simulink model "R2RSystemModel"  (R2014a)
settings: Solver=ode45  StartTime=StartTime  StopTime=StopTime  MaxStep=MaxStepSize  RelTol=1e-3
values from neighbouring files (symbols this model uses):
  ContactPoint = 23    [ControlDesign.m]
  Home = 0    [ControlDesign.m]
  K_L12_Force = 2.29181    [ControlDesign.m]    (also in ControlDesignForceModeLinear.m)
  K_PWM = PWM_res/V_rail    (= 83.3333333333)    [ControlDesign.m]    (also in ControlDesignForceModeLinear.m = 0.012)
  Kspring = 55    [ControlDesign.m]    (also in ControlDesignForceModeLinear.m = 100)
  L12_Offset_I = 12.995    [ControlDesign.m]    (also in ControlDesignForceModeLinear.m)
  PWM_res = 2000    [ControlDesign.m]    (also in ControlDesignForceModeLinear.m)
  Ra_L12 = 60    [ControlDesign.m]    (also in ControlDesignForceModeLinear.m)
libraries: simulink x2
settings Model: Creator=oberstare  LastModifiedBy=oberstar

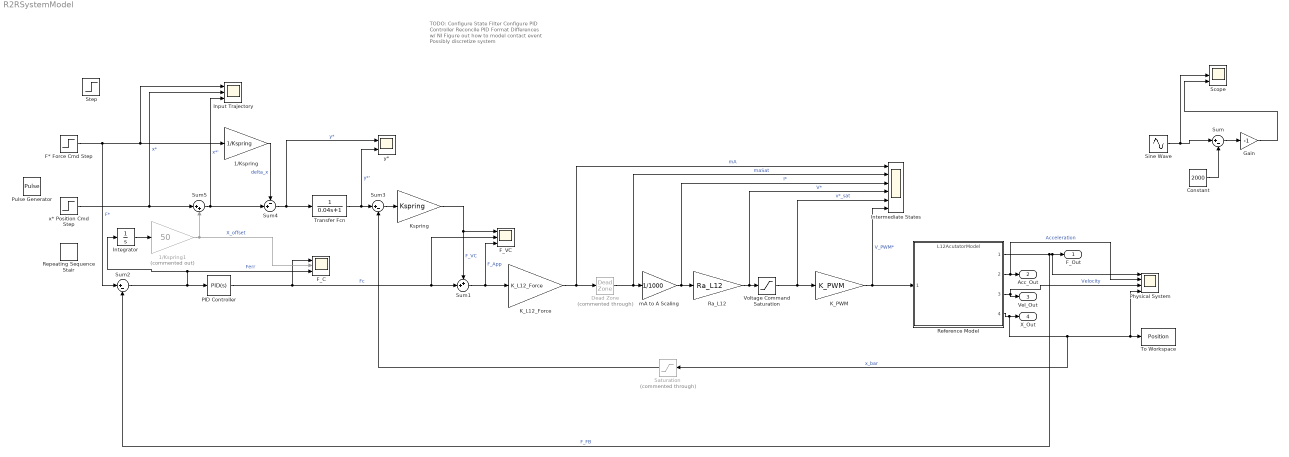
== system R2RSystemModel ==
  note: TODO:
      | Configure State Filter
      | Configure PID Controller
      | Reconcile PID Format Differences w/ NI
      | Figure out how to model contact event
      | Possibly discretize system
  1/Kspring : Gain  Gain=1/Kspring
  1/Kspring1 : Gain  Commented=on  Gain=50
  Constant : Constant  Value=2000
  Dead Zone : DeadZone  Commented=through  LowerValue=-1000/L12_Offset_I  UpperValue=1000/L12_Offset_I  SaturateOnIntegerOverflow=on
  F* Force Cmd Step : Step  Time=10  After=5  SampleTime=0
  F_C : Scope  NumInputPorts=3
      settings: YMin=-0.14~-5~-5  YMax=0.01~5~5  SaveName=ScopeData2
  F_VC : Scope  NumInputPorts=3
      settings: YMin=0~-0.15~0  YMax=1750~0.025~1750
  Gain : Gain  Gain=-1
  "Input Trajectory " : Scope  NumInputPorts=3
      settings: YMin=-1~0~0  YMax=1~30~35  SaveName=ScopeData3
  Integrator : Integrator
  Intermediate States : Scope  NumInputPorts=6
      settings: YMin=0~0~0~0~0~-5  YMax=4000~4000~4~225~2250~5  SaveName=ScopeData5
  K_L12_Force : Gain  Gain=K_L12_Force
  K_PWM : Gain  Gain=K_PWM
  Kspring : Gain  Gain=Kspring
  PID Controller : simulink/Continuous/PID Controller  Controller=PID  TimeDomain=Continuous-time  SampleTime=1  IntegratorMethod=Forward Euler  FilterMethod=Forward Euler  Form=Parallel  P=Kspring  I=0  D=0  N=100  InitialConditionSource=internal  InitialConditionForIntegrator=0  InitialConditionForFilter=0  ExternalReset=none  LimitOutput=off  UpperSaturationLimit=inf  LowerSaturationLimit=-inf  LinearizeAsGain=on  AntiWindupMode=none  Kb=1  TrackingMode=off  Kt=1  PParamMin=[]  PParamMax=[]  IParamMin=[]  IParamMax=[]  DParamMin=[]  DParamMax=[]  NParamMin=[]  NParamMax=[]  KbParamMin=[]  KbParamMax=[]  KtParamMin=[]  KtParamMax=[]  POutMin=[]  POutMax=[]  IOutMin=[]  IOutMax=[]  DOutMin=[]  DOutMax=[]  NOutMin=[]  NOutMax=[]  KbOutMin=[]  KbOutMax=[]  KtOutMin=[]  KtOutMax=[]  IntegratorOutMin=[]  IntegratorOutMax=[]  FilterOutMin=[]  FilterOutMax=[]  SumOutMin=[]  SumOutMax=[]  SumI1OutMin=[]  SumI1OutMax=[]  SumI2OutMin=[]  SumI2OutMax=[]  SumI3OutMin=[]  SumI3OutMax=[]  SumDOutMin=[]  SumDOutMax=[]  SaturationOutMin=[]  SaturationOutMax=[]  IntegratorContinuousStateAttributes=''  IntegratorStateMustResolveToSignalObject=off  IntegratorRTWStateStorageClass=Auto  FilterContinuousStateAttributes=''  FilterStateMustResolveToSignalObject=off  FilterRTWStateStorageClass=Auto
  Physical System : Scope  NumInputPorts=4
      settings: YMin=0~-4.5~-0.005~0  YMax=0.14~2~0.007~25  SaveName=ScopeData4
  Pulse Generator : DiscretePulseGenerator  PulseType=Time based  Amplitude=30  Period=20  PulseWidth=50  PhaseDelay=5
  Ra_L12 : Gain  Gain=Ra_L12
  Reference Model : ModelReference  ModelNameDialog=L12AcutatorModel.slx  SimulationMode=Normal  ModelReferenceVersion=1.67  CopyOfModelName=L12AcutatorModel.slx  DefaultDataLogging=on
  Repeating Sequence Stair : simulink/Sources/Repeating Sequence Stair  OutValues=[3 1 4 2 1].'  tsamp=-1  OutMin=[]  OutMax=[]  OutDataTypeStr=double  OutputDataTypeScalingMode=double  OutDataType=fixdt(0,8)  ConRadixGroup=Best Precision: Vector-wise  OutScaling=2^-12
  Saturation : Saturate  Commented=through  UpperLimit=ContactPoint  LowerLimit=Home
  Scope : Scope  NumInputPorts=3
      settings: YMin=-5~-5~-5  YMax=5~5~5  SaveName=ScopeData7
  Sine Wave : Sin  Amplitude=PWM_res  Bias=PWM_res  Phase=pi/2  SampleTime=0
  Step : Step  SampleTime=0
  Sum : Sum  Inputs=|+-
  Sum1 : Sum  Inputs=++|
  Sum2 : Sum  Inputs=|+-
  Sum3 : Sum  Inputs=|+-
  Sum4 : Sum  Inputs=-+|
  Sum5 : Sum  Inputs=|++
  To Workspace : ToWorkspace  VariableName=Position  SaveFormat=Timeseries  SampleTime=-1
  Transfer Fcn : TransferFcn  Denominator=[0.04 1]
  Voltage Command Saturation : Saturate  UpperLimit=12  LowerLimit=-12
  mA to A Scaling : Gain  Gain=1/1000
  x* Position Cmd Step : Step  After=22.5  SampleTime=0
  y* : Scope  NumInputPorts=2
      settings: YMin=0~0  YMax=35~35
  F_Out : Outport
  Acc_Out : Outport  Port=2
  Vel_Out : Outport  Port=3
  X_Out : Outport  Port=4
  wires:
  Reference Model/1 -> Physical System/1, F_Out/1, Sum2/2  "F_FB"
  Reference Model/2 -> Physical System/2, Acc_Out/1  "Acceleration"
  Reference Model/3 -> Physical System/3, Vel_Out/1  "Velocity"
  Constant/1 -> Sum/2
  Sum/1 -> Gain/1
  Gain/1 -> Scope/3
  Sine Wave/1 -> Scope/2, Sum/1
  Reference Model/4 -> Physical System/4, To Workspace/1, Saturation/1, X_Out/1  "x_bar"
  K_PWM/1 -> Intermediate States/6, Reference Model/1  "V_PWM*"
  mA to A Scaling/1 -> Intermediate States/3, Ra_L12/1  "I*"
  Dead Zone/1 -> Intermediate States/2, mA to A Scaling/1  "maSat"
  K_L12_Force/1 -> Dead Zone/1, Intermediate States/1  "mA"
  Sum1/1 -> F_VC/3, K_L12_Force/1  "F_App"
  Kspring/1 -> F_VC/1, Sum1/1  "F_VC"
  Sum3/1 -> Kspring/1
  F* Force Cmd Step/1 -> 1/Kspring/1, "Input Trajectory "/1, Sum2/1  "F*"
  1/Kspring/1 -> Sum4/1  "delta_x"
  Sum2/1 -> Integrator/1, F_C/3, PID Controller/1  "Ferr"
  PID Controller/1 -> F_C/1, F_VC/2, Sum1/2  "Fc"
  x* Position Cmd Step/1 -> Sum5/1, "Input Trajectory "/2  "x*"
  1/Kspring1/1 -> F_C/2, Sum5/2  "X_offset"
  Sum5/1 -> Sum4/2, "Input Trajectory "/3  "x*'"
  Transfer Fcn/1 -> y*/2, Sum3/1  "y*'"
  Sum4/1 -> Transfer Fcn/1, y*/1  "y*"
  Saturation/1 -> Sum3/2
  Voltage Command Saturation/1 -> Intermediate States/5, K_PWM/1  "v*_sat"
  Integrator/1 -> 1/Kspring1/1
  Ra_L12/1 -> Intermediate States/4, Voltage Command Saturation/1  "V*"
